simulink model "StateSpaceIntegralSLX"  (R2021a)
settings: Solver=VariableStepAuto  StartTime=0.0  StopTime=10.0  RelTol=1e-3
values from neighbouring files (symbols this model uses):
  K = K_amp(1:3)    [plantilla_sscontrol.m]
  L = minreal(P*C)    [plantilla.m]
undefined symbols (not defined in the file or in its folder): G, kI
settings Model: Creator=aghersin  LastModifiedBy=frand
settings SolverCC: AlgebraicLoopSolver=TrustRegion
settings DataIOCC: ReturnWorkspaceOutputs=off
settings DebuggingCC: SFMachineParentedDataDiag=warning  ArithmeticOperatorsInVariantConditions=warning
settings SFSimCC: SimUseLocalCustomCode=off  CustomCodeUndefinedFunction=UseInterfaceOnly
settings RTWCC: RTWUseLocalCustomCode=off

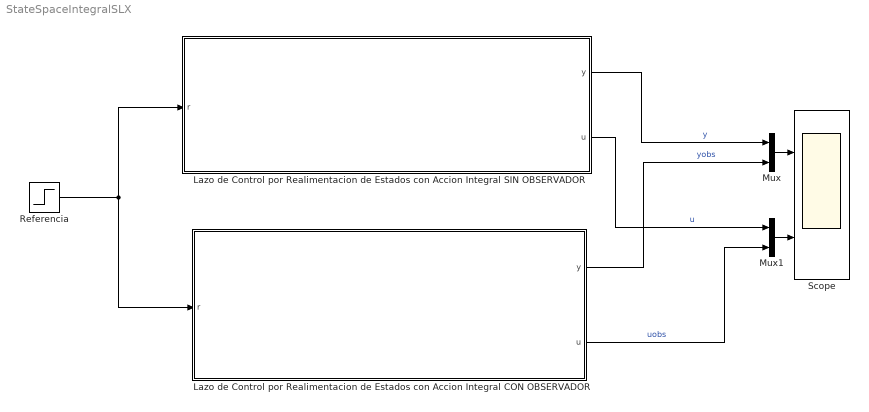
== system StateSpaceIntegralSLX ==
  Lazo de Control por Realimentacion de Estados con Accion Integral CON OBSERVADOR : Subsystem
  Lazo de Control por Realimentacion de Estados con Accion Integral SIN OBSERVADOR : Subsystem
  Mux : Mux  Inputs=2
  Mux1 : Mux  Inputs=2
  Referencia : Step  SampleTime=0
  Scope : Scope  NumInputPorts=2
  wires:
  Referencia/1 -> Lazo de Control por Realimentacion de Estados con Accion Integral CON OBSERVADOR/1(r), Lazo de Control por Realimentacion de Estados con Accion Integral SIN OBSERVADOR/1(r)
  Mux/1 -> Scope/1
  Mux1/1 -> Scope/2
  Lazo de Control por Realimentacion de Estados con Accion Integral SIN OBSERVADOR/1(y) -> Mux/1  "y"
  Lazo de Control por Realimentacion de Estados con Accion Integral SIN OBSERVADOR/2(u) -> Mux1/1  "u"
  Lazo de Control por Realimentacion de Estados con Accion Integral CON OBSERVADOR/1(y) -> Mux/2  "yobs"
  Lazo de Control por Realimentacion de Estados con Accion Integral CON OBSERVADOR/2(u) -> Mux1/2  "uobs"

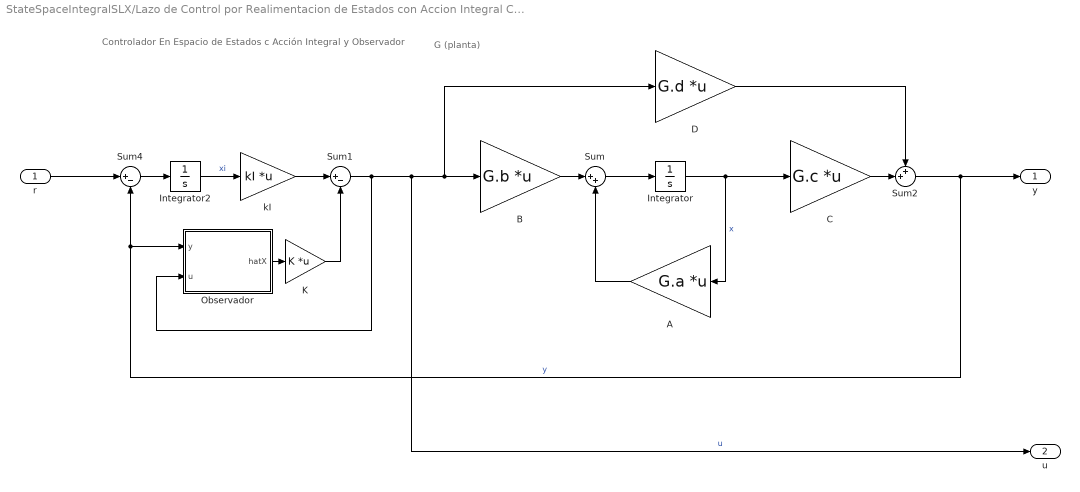
== system StateSpaceIntegralSLX/Lazo de Control por Realimentacion de Estados con Accion Integral CON OBSERVADOR ==
  note: Controlador
      | En Espacio de
      | Estados c
      | Acción Integral
      | y Observador
  note: G (planta)
  r : Inport
  A : Gain  Gain=G.a  Multiplication=Matrix(K*u)
  B : Gain  Gain=G.b  Multiplication=Matrix(K*u)
  C : Gain  Gain=G.c  Multiplication=Matrix(K*u)
  D : Gain  Gain=G.d  Multiplication=Matrix(K*u)
  Integrator : Integrator  InitialCondition=[1;2]
  Integrator2 : Integrator
  K : Gain  Gain=K  Multiplication=Matrix(K*u)
  Observador : Subsystem
  Sum : Sum  Inputs=|++
  Sum1 : Sum  Inputs=|+-
  Sum2 : Sum  Inputs=++|
  Sum4 : Sum  Inputs=|+-
  kI : Gain  Gain=kI  Multiplication=Matrix(K*u)
  y : Outport  VectorParamsAs1DForOutWhenUnconnected=off
  u : Outport  Port=2  VectorParamsAs1DForOutWhenUnconnected=off
  wires:
  Integrator/1 -> A/1, C/1  "x"
  C/1 -> Sum2/2
  Sum/1 -> Integrator/1
  D/1 -> Sum2/1
  A/1 -> Sum/2
  B/1 -> Sum/1
  K/1 -> Sum1/2
  Sum4/1 -> Integrator2/1
  r/1 -> Sum4/1
  Observador/1(hatX) -> K/1
  Sum1/1 -> B/1, D/1, u/1, Observador/2(u)  "u"
  Sum2/1 -> Sum4/2, Observador/1(y), y/1  "y"
  Integrator2/1 -> kI/1  "xi"
  kI/1 -> Sum1/1

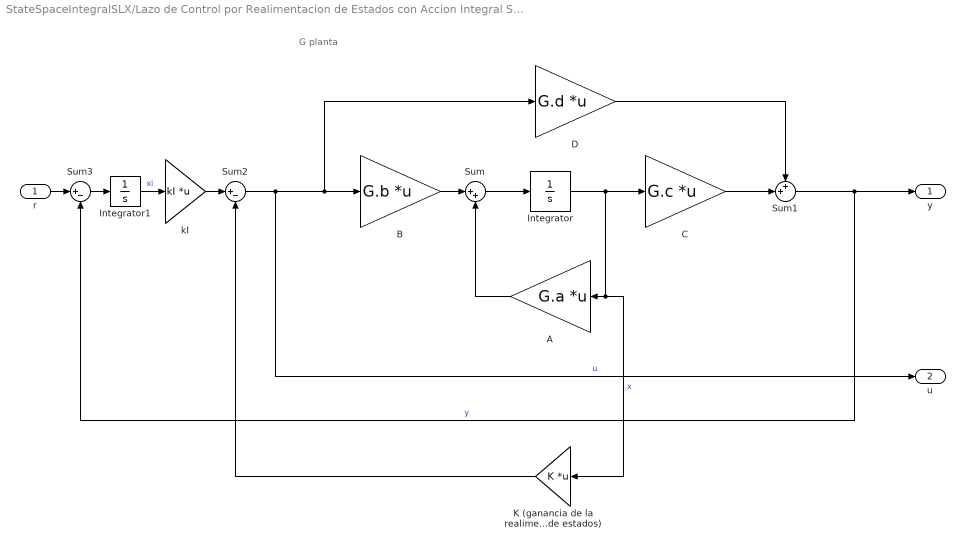
== system StateSpaceIntegralSLX/Lazo de Control por Realimentacion de Estados con Accion Integral SIN OBSERVADOR ==
  note: G
      | planta
  r : Inport
  A : Gain  Gain=G.a  Multiplication=Matrix(K*u)
  B : Gain  Gain=G.b  Multiplication=Matrix(K*u)
  C : Gain  Gain=G.c  Multiplication=Matrix(K*u)
  D : Gain  Gain=G.d  Multiplication=Matrix(K*u)
  Integrator : Integrator  InitialCondition=[1;2]
  Integrator1 : Integrator
  K (ganancia de la realimentacion de estados) : Gain  Gain=K  Multiplication=Matrix(K*u)
  Sum : Sum  Inputs=|++
  Sum1 : Sum  Inputs=++|
  Sum2 : Sum  Inputs=|+-
  Sum3 : Sum  Inputs=|+-
  kI : Gain  Gain=kI  Multiplication=Matrix(K*u)
  y : Outport  VectorParamsAs1DForOutWhenUnconnected=off
  u : Outport  Port=2  VectorParamsAs1DForOutWhenUnconnected=off
  wires:
  Integrator/1 -> K (ganancia de la realimentacion de estados)/1, A/1, C/1  "x"
  Integrator1/1 -> kI/1  "xi"
  Sum1/1 -> y/1, Sum3/2  "y"
  kI/1 -> Sum2/1
  K (ganancia de la realimentacion de estados)/1 -> Sum2/2
  Sum3/1 -> Integrator1/1
  Sum2/1 -> u/1, D/1, B/1  "u"
  r/1 -> Sum3/1
  B/1 -> Sum/1
  A/1 -> Sum/2
  D/1 -> Sum1/1
  Sum/1 -> Integrator/1
  C/1 -> Sum1/2

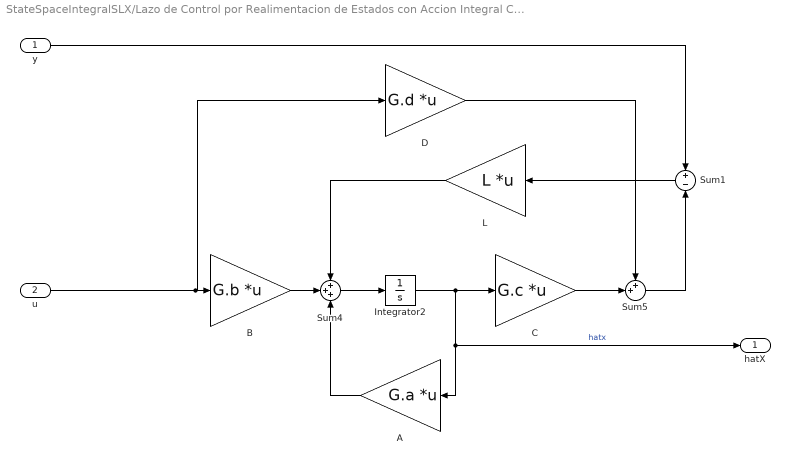
== system StateSpaceIntegralSLX/Lazo de Control por Realimentacion de Estados con Accion Integral CON OBSERVADOR/Observador ==
  y : Inport
  u : Inport  Port=2
  A : Gain  Gain=G.a  Multiplication=Matrix(K*u)
  B : Gain  Gain=G.b  Multiplication=Matrix(K*u)
  C : Gain  Gain=G.c  Multiplication=Matrix(K*u)
  D : Gain  Gain=G.d  Multiplication=Matrix(K*u)
  Integrator2 : Integrator
  L : Gain  Gain=L  Multiplication=Matrix(K*u)
  Sum1 : Sum  Inputs=+|-
  Sum4 : Sum  Inputs=+++
  Sum5 : Sum  Inputs=++|
  hatX : Outport  VectorParamsAs1DForOutWhenUnconnected=off
  wires:
  L/1 -> Sum4/1
  A/1 -> Sum4/3
  B/1 -> Sum4/2
  u/1 -> D/1, B/1
  Sum4/1 -> Integrator2/1
  C/1 -> Sum5/2
  D/1 -> Sum5/1
  Sum1/1 -> L/1
  Integrator2/1 -> C/1, A/1, hatX/1  "hatx"
  Sum5/1 -> Sum1/2
  y/1 -> Sum1/1
